simulink library "FPGA_Open_Speech_Tools"  (R2020b)
settings: Solver=VariableStepAuto  StartTime=0.0  StopTime=10.0  RelTol=1e-3
undefined symbols (not defined in the file or in its folder): a, b, c, tableInit
libraries: hdlsllib x159, simulink x26, $bdroot x3
(part 1 of 4)
settings Model: Creator=E. Bailey Galacci  LastModifiedBy=conno
settings SFSimCC: CustomCodeUndefinedFunction=UseInterfaceOnly

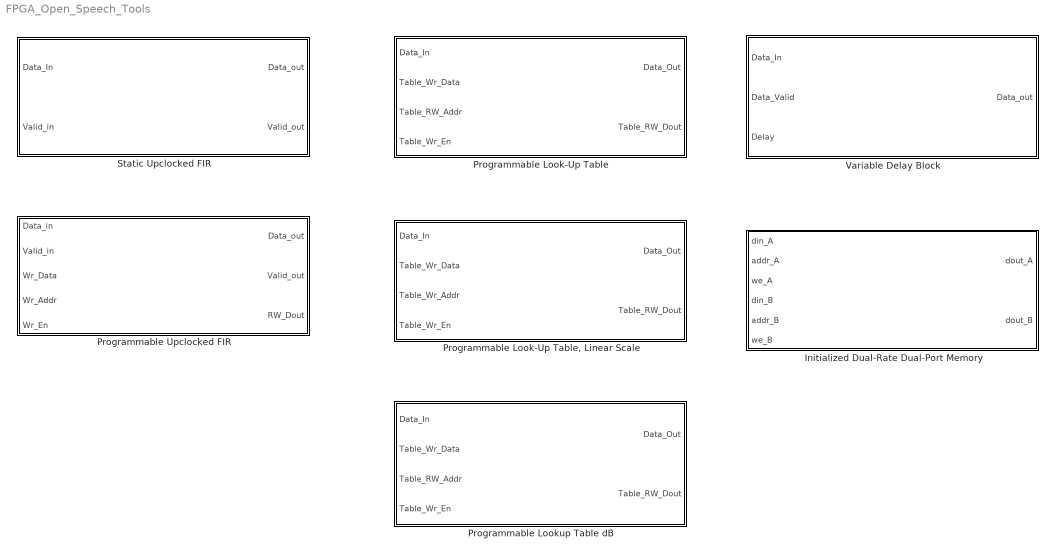
== system FPGA_Open_Speech_Tools ==
  Initialized Dual-Rate Dual-Port Memory : Subsystem  mask(Dual-rate dual-port RAM){ram_size=8, Table_Init=tableInit}
      mask prompts: ram_size "Address port width (2 to 29 bits)"; Table_Init "Table Initialized Values (vector)"
      mask help: This block simulates a dual-clock dual-port RAM with two data output ports. The memory is initialized with values from the Table_Init input vector.
      mask init:
      | hdlblkmask_drdpram;
      mask Help: helpview([docroot '/hdlcoder/helptargets.map'],'HDL_dual_rate_dual_port_ram');
      mask Display:
      | disp(sprintf(['Initialized Dual-Rate \n Dual-Port Memory']));
      | port_label('input',1,'din_A');
      | port_label('input',2,'addr_A');
      | port_label('input',3,'we_A');
      | port_label('input',4,'din_B');
      | port_label('input',5,'addr_B');
      | port_label('input',6,'we_B');
      | port_label('output',1,'dout_A');
      | port_label('output',2,'dout_B');
  Programmable Look-Up Table : Subsystem  mask(Programmable Look-Up Table){tableFnParam=xIn.^0.5, SAVE_TABLE=off, maxInput=1, floorParam=2^-15, errorParam=.1, ERR_DIAG=off, PLOT_TABLE=off, nBitsParam=4, mBitsParam=5, IGOTTHIS=off, W_bits=32, F_bits=28, tableInit=0, binaryOffset=0}
      mask prompts: tableFnParam "Table Represented Function"; SAVE_TABLE "Save Table Input/Output set as .mat"; maxInput "Maximum Input Value"; floorParam "Minimum Input Threshold"; errorParam "Maximum Allowed Error (%)"; ERR_DIAG "Show Error Calculation"; PLOT_TABLE "Show Table Init Plot"; nBitsParam "N_bits"; mBitsParam "M_bits"; IGOTTHIS "Manual Bit Definition Override"; W_bits "Word Bits"; F_bits "Fractional Bits"
      mask help:
      | A hardware-oriented implementation of a lookup table.
      | Provides a fairly resource efficient way to avoid hardware-difficult operations, such as logarithms or square roots.
      | Tables can be initialized on system startup and rewritten during runtime using the Table_Wr lines.
      | Min input cannot be 0, because inputs are pseudo-logarithmically spaced.
      |
      | Input and Output set can be saved as "xIn" and "tableInit" within the file "<path name> init.mat". Input values remain constant
      | until the mask parameters are updated. Table Output values can be reprogrammed during runtime using the Wr_Data, Wr_En and RW_Addr lines.
      mask init:
      | %% PLUT INIT SCRIPT
      | %
      | % This script is a copy of code used in the Programmable Look-Up Table's
      | % init script in the DSP_FPGA_Accelerated_Toolbox.
      | 
      | % Copyright 2020 Flat Earth Inc
      | %
      | % THE SOFTWARE IS PROVIDED "AS IS", WITHOUT WARRANTY OF ANY KIND, EXPRESS OR IMPLIED,
      | % INCLUDING BUT NOT LIMITED TO THE WARRANTIES OF MERCHANTABILITY, FITNESS FOR A PARTICULAR
      | % PURPOSE AND NONINFRINGEMENT. IN NO EVENT SHALL THE AUTHORS OR COPYRIGHT HOLDERS BE LIABLE
      | % FOR ANY CLAIM, DAMAGES OR OTHER LIABILITY, WHETHER IN AN ACTION OF CONTRACT, TORT OR OTHERWISE,
      | % ARISING FROM, OUT OF OR IN CONNECTION WITH THE SOFTWARE OR THE USE OR OTHER DEALINGS IN THE SOFTWARE.
      | %
      | % E. Bailey Galacci
      | % Flat Earth Inc
      | % 985 Technology Blvd
      | % Bozeman, MT 59718
      | % support@flatearthinc.com
      | 
      | % things to display: table size, input bounds, function, accuracy
      | % things to figure out: M_bits, N_bits, Min_val, X_in table, Y_out table,
      | % max_error, ram_size, table_size 
      | 
      | binaryOffset = ceil(log2(maxInput)); % used for binary tricks, as well as identifying input range
      | if(IGOTTHIS)
      |     N_bits = nBitsParam;
      |     M_bits = mBitsParam;
      | else
      |     N_bits = ceil(log2(binaryOffset-log2(floorParam)+1));
      |     % M_bits needs to be defined later, as it must be just enough to meet
      |     % accuracy standards defined by user, with linear interpolation
      |     M_bits = 1; %this will be updated later as needed
      | end
      | 
      | repeatFlag = true;
      | while(repeatFlag)
      |     % Define a N point log2 spaced range of inputs, from 2^(d-(2^N_bits -1)) to almost 2^(d+1), 
      |     % this effectively covers the user defined input range, down to a floor
      |     % value.
      |     xIn = zeros(1, 2^(M_bits+N_bits));
      |     addr = 1;
      |     for NShifts = 2^N_bits-1:-1:0
      |         for M = 0:2^M_bits - 1
      |             xIn(addr) = 2^(binaryOffset-NShifts) + M*2^(binaryOffset-NShifts-M_bits);
      |             addr = addr+1;
      |         end
      |     end
      | 
      |     % use function to define output. note: function must contain input xIn
      |     % within the string to work properly, and the only output of the function
      |     % must be the table values.
      |     tableInit = eval(tableFnParam);
      | 
      |     RAM_SIZE = N_bits+M_bits;
      |     maxVal = 2^binaryOffset+ (2^M_bits -1)*2^(binaryOffset-M_bits);
      |     minVal = 2^(binaryOffset-(2^N_bits-1));
      |     %set_param(gcb,'MaskDisplay',"disp(sprintf('Programmable Look-up Table\nMemory Used = %d samples and coeffs\nClock Rate Needed = %d Hz', FIR_Uprate*2, Max_Rate)); port_label('input',1,'data'); port_label('input',2,'valid'); port_label('input',3,'Wr_Data'); port_label('input',4,'Wr_Addr'); port_label('input',5,'Wr_En'); port_label('output',1,'data'); port_label('output',2,'valid'); port_label('output',3,'RW_Dout');")
      | 
      |     %%%%%%%%%% check and identify error %%%%%%%%%%%
      |     % Define a set of test cases for the lookup table with log spaced points
      |     xTest = logspace(log10(minVal), log10(maxVal), 2^(RAM_SIZE+2));
      |     xTemp = xIn;
      |     xIn = xTest;
      |     % identify the values of the function at xTest
      |     yTest = eval(tableFnParam);
      | 
      |     % move lookup table input values back to xIn
      |     xIn = xTemp;
      | 
      |     % Find lookup addresses for each point in xTest
      |     % Effectively assumes the highest input value, then decreases address until test input is greater than associated table input at that address
      |     addrTest = zeros(1,length(xTest));
      |     for it = 1:length(xTest)
      |         addrTest(it) = 2^RAM_SIZE;
      |         while(xTest(it) < xIn(addrTest(it)) && addrTest(it) ~= 1)   % find the address associated with an input value closest to and below xTest
      |             addrTest(it) = addrTest(it) - 1;
      |         end
      |         if(addrTest(it)==0)
      |             addrTest(it) = 1;
      |         end
      |     end
      | 
      |     % Check for any possible out of bounds errors (handled similarly in hardware)
      |     addrTest(addrTest == 2^RAM_SIZE) = 2^RAM_SIZE -1;
      | 
      |     % Get values for linear interpolation of xIn
      |     xLow  = xIn(addrTest);
      |     xHigh = xIn(addrTest+1);
      | 
      |     % apply point-slope formula to preform linear interpolation for the table readout
      |     yLow  = tableInit(addrTest);
      |     yHigh = tableInit(addrTest+1);
      |     slope  = (yHigh-yLow) ./ (xHigh - xLow);
      |     yInter = slope.*(xTest-xLow)+yLow;
      |     
      |     % percent error: obt-exp / exp
      |     %errorFloor = (yTest-yLow)./yTest;  % w/out linear interpolation
      |     errorInter = (yTest-yInter)./yTest; % w/ linear interpolation
      |     maxErr = max(abs(errorInter));
      |     %check while loop condition
      |     if(IGOTTHIS) 
      |         repeatFlag = false;
      |     else
      |         if(100*maxErr <= abs(errorParam))
      |             repeatFlag = false;
      |         else
      | %             if(ERR_DIAG)
      | %                 f = msgbox(sprintf('Err = %.2d, M_bits = %d', 100*maxErr, M_bits),'Configuring PLUT','replace');
      | %             end
      |             
      |             % make table larger to increase accuracy. M_bits can increase
      |             % by more than 1 to save loops if error is far outside bounds
      |             if(100*maxErr > 8*errorParam)
      |                 M_bits = M_bits+3;
      |             elseif(100*maxErr > 4*errorParam)
      |                 M_bits = M_bits+2;
      |             else
      |                 M_bits = M_bits+1;
      |             end
      |         end
      |     end
      | end%end while loop
      | % prinout graph of table values and error test
      | if(ERR_DIAG)
      |     figure(1); 
      |     f = msgbox(sprintf('%s\nErr = %.2d %%, Ram Size = %d bits  (2 by %d by %d)\n Address Width: %d, N_bits: %d, M_bits: %d', gcb, 100*maxErr, 2*2^RAM_SIZE*W_bits, 2^RAM_SIZE, W_bits, RAM_SIZE, N_bits, M_bits), sprintf('PLUT INIT: %s', gcb),'replace');
      |     subplot(2,1,1); semilogx(xTest,yInter, xTest,yTest,xIn,tableInit,'k*'); title('Output Values over Input Range'); xlabel('Inputs'); ylabel('Outputs'); legend('Interpolated Results','Ideal','Table Points');
      |     subplot(2,1,2); semilogx(xTest,100*errorInter); title('Error of Output over Input Range'); xlabel('Inputs'); ylabel('Percent Error');
      | end
      | 
      | % Some testing variables. Uncomment if desired.
      | %maxFloorErrTot = max(maxFloorErr);
      | %maxInterErrTot = max(maxInterErr);
      | 
      | % Plot the LUT's inital table set
      | if(PLOT_TABLE)
      |     % Handle String errors? 
      |     figure(2); semilogx(xIn,tableInit, 'k*'); title(sprintf('Table Initialized Function: %s', tableFnParam),'Interpreter','none');
      | end 
      | % Save Input and Output set to a .mat file
      | if(SAVE_TABLE)
      |     fileName = [gcb '_init'];
      |     fileName(fileName == '/') = '_'; % Replace slashes with underscores
      |     address = 0:(2^RAM_SIZE)-1;
      |     save(fileName, 'xIn', 'address', 'tableInit');
      | end
      | set_param(gcb,'MaskDisplay',"disp(sprintf(['Programmable Look-Up Table\nMemory Used: %d bits, Address Width: %d\n' tableFnParam ': %.2d <= x <= %.2d\n Maximum Error: %.2d %%'], 2*2^RAM_SIZE*W_bits, RAM_SIZE, minVal, maxVal, 100*maxErr)); port_label('input',1,'Data_In'); port_label('input',2,'Table_Wr_Data'); port_label('input',3,'Table_RW_Addr'); port_label('input',4,'Table_Wr_En'); port_label('output',1,'Data_Out'); port_label('output',2,'Table_RW_Dout');")
      mask Help:
      | A hardware-oriented implementation of a lookup table.
      | Provides a fairly resource efficient way to avoid hardware-difficult operations, such as logarithms or square roots.
      | Tables can be initialized on system startup and rewritten during runtime using the Table_Wr lines.
      | Min input cannot be 0, because inputs are pseudo-logarithmically spaced.
      | 
      | Input and Output set can be saved as "xIn" and "tableInit" within the file "<path name> init.mat". Input values remain constant
      | until the mask parameters are updated. Table Output values can be reprogrammed during runtime using the Wr_Data, Wr_En and RW_Addr lines.
      | 
      | Uses pseudo-logarithmic spacing of inputs for maximum accuracy in non-linear functions, as well as linear interpolation between points to further increase accuracy. Because of this, it is assumed that function input is unsigned. If this is undesired, a second table would need to be implemented to cover negative values, or some other solution outside the block.
      | 
      | Capable of automatically determining required table size to meet a given accuracy requirement within the entire data range, or can be manually set to a specific size with M_bits and N_bits. N_bits determines the data range as a power of 1/2 of the maximum input. M_bits determines the number of bits in the address used to increase function precision, by increasing the number of points stored between each log2 spaced input point.
      | 
      | 
      | 
      | ------------------
      | Mask Parameters
      | ------------------
      | 
      | Table Represented Function:
      |   Function to estimate using the lookup table. Must contain the variable "X_in" as an input to a function, or as a variable within the executable code string, as this is used in the Initialization code to evaluate the function. If a function, that function must also have a single output which will define the values to fill the table with given input value X_in.
      | 
      | Save Table Input/Output set as .mat
      |   If asserted, the table's inputs and outputs will be saved in a .mat file named "<path name>_init.mat". By loading this, it is possible to see all precalculated points of the look-up table. This is especially useful when trying to reprogram the table, as all input points are shown along with their associated addresses.
      | 
      | --Table Parameters--
      |   Maximum Input Value:
      |     The maximum input value the table should be expected to represent. If the input value is greater than this parameter's nearest higher power of 2, the table will output the value for the highest input.
      | 
      | --Define Input Threshold and Accuracy Tab--
      |   Minimum Input Threshold:
      |     The minimum input to recognize by the table. If the input value is less than this parameter's the nearest lower power of 2, the table will output the value for the lowest input.
      | 
      |   Maximum Allowed Error (%):
      |     The amount of percent error allowed by the table. Used by the init script to identify the size of the table required to meet this parameter. This is found by testing a set of examples 4 times larger than the table set, therefore it is possible on rare occasion for some points to exceed this error. Decreasing this will increase the memory required for the table, but increase precision.
      | 
      |   Show Error Calculation:
      |     When asserted, the block will show a figure of the error calculation and a pop-up detailing the amount of memory used, size of the RAM allocated, and maximum error.
      | 
      |   Show Table Init Plot:
      |     When asserted, the block will show a figure of the table's initialized values.
      | 
      | --Define Address Space Manually Tab--
      |   N_bits:
      |     Only used when Manual Bit Definition Override is asserted.
      |     The width of the address dedicated to breadth of valid data. Increasing this will cause the table to recognize smaller numbers (by increasing the size of the Leading Zero Counter's output)  at the cost of memory used, and more logic required in the LZC.
      |   M_bits:
      |     Only used when Manual Bit Definition Override is asserted.
      |     The width of the address dedicated to depth of valid data. Increasing this will cause more bits of the input to be considered as part of the address after the Leading Zero Counter, increasing precision at the cost of memory.
      | 
      |   Manual Bit Definition Override:
      |     Checking this box will skip automatic size definition of Leading Zero Counter and precision bit size. Use with caution, as percent error will not be guaranteed with this setting on. Read the formal documentation for more details, kept within the file structure this library is stored in.
      | 
      | 
      | --Data Parameters dropdown--
      | Word Bits:
      |   Size of fixed point word of both the input signal and table memory.
      | 
      | Fractional Bits:
      |   Number of fractional bits in the fixed point word of both the input signal and table memory.
      | 
      | ----------
      | Block I/O
      | ----------
      | INPUTS:
      | 
      | --Data_In--
      |   Input signal to be looked-up. Expected size fixdt(0,Word Bits, Fractional Bits).
      | 
      | --Table_Wr_Data-- % Table Write Data
      |   Data to write to the table, in location Table_RW_Addr, when Table_Wr_En is asserted. Expected size fixdt(0,Word Bits, Fractional Bits).
      | 
      | --Table_RW_Addr-- % Table Read/Write Address
      |   The location within the table to read or overwrite. Expected size changes based on the function and allowed error as initialized, and is shown on the Mask Label as RAM Width, or by checking the "Show Error Calculation" button as RAM Width.
      |   There is an internal check that will correct a signal of the wrong size to the correct address size, but it may be useful to know the X values associated with table output at any given address. Using the "Save Table Input/Output as .mat" option will save the entire set of initialized inputs and outputs along with their associated addresses.
      |   For a full explanation on how xIn is derived, see the formal documentation contained within the file structure this library is stored in.
      | 
      | --Table_Wr_En-- % Table Write Enable
      |   Boolean. If this line is asserted, address Table_RW_Addr will be overwritten with data Table_Wr_Data.
      | 
      | 
      | OUTPUTS:
      | --Data_Out--
      |   Output data of the table. Size fixdt(1,Word Bits, Fractional Bits).
      | 
      | --Table_RW_Dout-- % Table Read/Write Data Out
      |   Outputs the data currently within address Table_RW_Addr (after writing if Table_Wr_En is asserted). Size fixdt(1, Word Bits, Fractional Bits).
      mask DialogControl Control2_copy Prompt: Must be a function of "xIn" to get table values
      mask DialogControl Container3 Prompt: Table Parameters
      mask DialogControl Container5 Prompt: Define Input Threshold and Accuracy
      mask DialogControl Container7 Prompt: Define Address Space Manually
      mask DialogControl Control2 Prompt: See Documentation for details
      mask DialogControl Container9 Prompt: Data Parameters
      mask Display: disp(sprintf(['Programmable Look-Up Table\nMemory Used: %d bits, Address Width: %d\n' tableFnParam ': %.2d <= x <= %.2d\n Maximum Error: %.2d %%'], 2*2^RAM_SIZE*W_bits, RAM_SIZE, minVal, maxVal, 100*maxErr)); port_label('input',1,'Data_In'); port_label('input',2,'Table_Wr_Data'); port_label('input',3,'Table_RW_Addr'); port_label('input',4,'Table_Wr_En'); port_label('output',1,'Data_Out'); port_label('output',2,'Table_RW_Dout');
  "Programmable Look-Up Table, Linear Scale" : Subsystem  mask(Programmable Look-Up Table){tableFnParam=sin(xIn), SAVE_TABLE=off, errorParam=.1, ERR_DIAG=off, PLOT_TABLE=off, ADDR_W_MANUAL=4, IGOTTHIS=off, W_bits=32, F_bits=28, isSigned=on, tableInit=0}
      mask prompts: tableFnParam "Table Represented Function"; SAVE_TABLE "Save Table Input/Output set as .mat"; errorParam "Maximum Allowed Error (+/-)"; ERR_DIAG "Show Error Calculation"; PLOT_TABLE "Show Table Init Plot"; ADDR_W_MANUAL "Address Width"; IGOTTHIS "Manual Bit Definition Override"; W_bits "Word Bits"; F_bits "Fractional Bits"; isSigned "Data Signed?"
      mask help:
      | A hardware-oriented implementation of a lookup table.
      | Provides a fairly resource efficient way to avoid hardware-difficult operations, such as logarithms or square roots.
      | Tables can be initialized on system startup and rewritten during runtime using the Table_Wr lines.
      mask init:
      | %% LINEAR PLUT INIT SCRIPT
      | 
      | % Copyright 2020 Flat Earth Inc
      | %
      | % THE SOFTWARE IS PROVIDED "AS IS", WITHOUT WARRANTY OF ANY KIND, EXPRESS OR IMPLIED,
      | % INCLUDING BUT NOT LIMITED TO THE WARRANTIES OF MERCHANTABILITY, FITNESS FOR A PARTICULAR
      | % PURPOSE AND NONINFRINGEMENT. IN NO EVENT SHALL THE AUTHORS OR COPYRIGHT HOLDERS BE LIABLE
      | % FOR ANY CLAIM, DAMAGES OR OTHER LIABILITY, WHETHER IN AN ACTION OF CONTRACT, TORT OR OTHERWISE,
      | % ARISING FROM, OUT OF OR IN CONNECTION WITH THE SOFTWARE OR THE USE OR OTHER DEALINGS IN THE SOFTWARE.
      | %
      | % E. Bailey Galacci
      | % Flat Earth Inc
      | % 985 Technology Blvd
      | % Bozeman, MT 59718
      | % support@flatearthinc.com
      | 
      | % things to display: table size, floor input?, max input, accuracy
      | % things to figure out: M_bits, N_bits, Min_val, X_in table, Y_out table,
      | % maxError, RAM_SIZE, table size 
      | 
      | if(IGOTTHIS)
      |     N_bits = ADDR_W_MANUAL;
      | else
      |     N_bits = 4;
      |     % N_bits will likely need to be updated later, until table is large enough to meet
      |     % accuracy standards defined by user
      | end;
      | 
      | repeatFlag = true;
      | while(repeatFlag)
      |     % Define a 2^N point log2 spaced range of inputs, from 2^(d-(2^N_bits -1)) to almost 2^(d+1), 
      |     % this effectively covers the user defined input range, down to a floor
      |     % value.
      |     % Signed vs Unsigned: If signed, treat word size as 1 smaller for max and
      |     % min inputs
      |     % Signed: 
      |     % smallest table input: -2^(W-1-F), 2's compliment, "[1, zeros(1,N-1)]"
      |     % step size: 2^(W-F-N)
      |     % largest table input: 2^(W-1-F) - 2^(W-F-N), smallest number but positive
      |     % and minus 1 step size, "[0, ones(1,N-1)]"
      |     % Unsigned: 
      |     % smallest table input: 0
      |     % step size: 2^(W-F-N)
      |     % largest table input: 2^(W-1-F) - 2^(W-F-N), smallest number but positive
      |     % and minus 1 step size, "[ones(1,N)]"
      |     if(isSigned)
      |         xIn = -2^(W_bits-1-F_bits) : 2^(W_bits-F_bits-N_bits) : 2^(W_bits-1-F_bits) - 2^(W_bits-F_bits-N_bits);
      |     else
      |         xIn = 0 : 2^(W_bits-F_bits-N_bits) : 2^(W_bits-F_bits) - 2^(W_bits-F_bits-N_bits);
      |     end
      | 
      |     % use function to define output. note: function must contain input xIn
      |     % within the string to work properly, and the only output of the function
      |     % must be Y_out.
      |     tableInit = eval(tableFnParam);
      | 
      |     RAM_SIZE = N_bits;
      |     maxVal = xIn(end);
      |     minVal = xIn(1);
      |     %set_param(gcb,'MaskDisplay',"disp(sprintf('Programmable Look-up Table\nMemory Used = %d samples and coeffs\nClock Rate Needed = %d Hz', FIR_Uprate*2, Max_Rate)); port_label('input',1,'data'); port_label('input',2,'valid'); port_label('input',3,'Wr_Data'); port_label('input',4,'Wr_Addr'); port_label('input',5,'Wr_En'); port_label('output',1,'data'); port_label('output',2,'valid'); port_label('output',3,'RW_Dout');")
      | 
      |     %%%%%%%%%% check and identify error %%%%%%%%%%%
      |     % Make some values for an "ideal" lookup table with lin spaced points
      |     if(isSigned)
      |         xTest = -2^(W_bits-1-F_bits) : 2^(W_bits-F_bits-N_bits-2) : 2^(W_bits-1-F_bits) - 2^(W_bits-F_bits-N_bits);
      |     else
      |         xTest = 0 : 2^(W_bits-F_bits-N_bits-2) : 2^(W_bits-F_bits) - 2^(W_bits-F_bits-N_bits);
      |     end
      |     xTemp = xIn;
      |     xIn = xTest;
      |     % identify the values of the function at xTest
      |     yTest = eval(tableFnParam);
      | 
      |     % Return table input set to xIn (already have xTemp)
      |     xIn = xTemp;
      | 
      |     % Find lookup addresses for each point in xTest
      |     addrTest = zeros(1,length(xTest));
      |     for it = 1:length(xTest)
      |         addrTest(it) = 2^RAM_SIZE;
      |         while(xTest(it) < xIn(addrTest(it)) && addrTest(it) ~= 1)
      |             addrTest(it) = addrTest(it) - 1;
      |         end
      |         if(addrTest(it)==0) %% sanity check for out of bounds results
      |             addrTest(it) = 1;
      |         end
      |     end
      |     
      |     yLow = tableInit(addrTest);
      | 
      |     % Check for any possible out of bounds errors (handled similarly in
      |     % hardware)
      |     addrTest(addrTest == 2^RAM_SIZE) = 2^RAM_SIZE -1;
      | 
      |     
      |     % absolute error: abs(obt-exp)
      |     errorFloor = abs(yTest-yLow);
      |     NAN_CLEANUP = isnan(errorFloor);
      |     errorFloor(NAN_CLEANUP) = 0;
      |     %errorInter = (Y_out_Ideal-y_inter)./Y_out_Ideal;
      |     %maxFloorErr(ix) = 100*max(abs(errorFloor(ix, 2870:9839)));
      |     %maxInterErr(ix) = 100*max(abs(errorInter(ix, 2870:9839)));
      |     maxErr = max(abs(errorFloor));
      |     
      |     %check while loop condition
      |     if(IGOTTHIS) 
      |         repeatFlag = false;
      |     end
      |     
      |     if(maxErr <= abs(errorParam) || N_bits > W_bits)
      |         repeatFlag = false;
      |     else
      | %        if(ERR_DIAG)
      | %            f = msgbox(sprintf('Err = %.2d, N_bits = %d', maxErr, N_bits),'Configuring PLUT','replace');
      | %        end
      |         
      |         % make table larger to increase accuracy
      |         if(maxErr > abs(errorParam))
      |             N_bits = N_bits+1;
      |         end
      |     end
      | end%end while loop
      | 
      | % Plot the LUT's inital table set
      | if(PLOT_TABLE)
      |     % Handle String errors? 
      |     figure(2); semilogx(xIn,tableInit, 'k*'); title(sprintf('Table Initialized Function: %s', tableFnParam),'Interpreter','none');
      | end 
      | 
      | % printout graph of table values and error test
      | if(ERR_DIAG)
      |     figure(1); 
      |     f = msgbox(sprintf('Err = +/- %.2d, Ram Size = %d bits  (%d by %d)', maxErr, 2^RAM_SIZE*W_bits, 2^RAM_SIZE, W_bits),gcb,'replace');
      |     subplot(2,1,1); plot(xTest,yLow, xTest,yTest,xIn,tableInit,'k*'); title('Output Values over Input Range'); xlabel('Inputs'); ylabel('Outputs'); legend('Table Results','Ideal','Table Points');
      |     subplot(2,1,2); plot(xTest, errorFloor); title('Error of Output over Input Range'); xlabel('Inputs'); ylabel('Absolute Error');
      | end
      | 
      | if(isSigned) % setup for 2's compliment
      |     tableInit = [tableInit(2^(N_bits-1)+1:end) , tableInit(1:2^(N_bits-1))];
      |     xInInit = [xIn(2^(N_bits-1)+1:end), xIn(1:2^(N_bits-1))];
      | else
      |     tableInit = tableInit;
      |     xInInit = xIn;
      | end
      | 
      | % Save Input and Output set to a .mat file
      | if(SAVE_TABLE)
      |     fileName = [gcb '_init'];
      |     fileName(fileName == '/') = '_'; % Replace slashes with underscores
      |     address = 0:(2^RAM_SIZE)-1;
      |     save(fileName, 'xInInit', 'address', 'tableInit');
      | end
      | 
      | set_param(gcb,'MaskDisplay',"disp(sprintf(['Programmable Look-Up Table\nMemory Used = %d bits, Address Width: %d\n' tableFnParam ': %d <= x <= %d \n Maximum Error: +/-%.2d'], 2^RAM_SIZE*W_bits, RAM_SIZE, minVal, maxVal, maxErr)); port_label('input',1,'Data_In'); port_label('input',2,'Table_Wr_Data'); port_label('input',3,'Table_RW_Addr'); port_label('input',4,'Table_Wr_En'); port_label('output',1,'Data_Out'); port_label('output',2,'Table_RW_Dout');")
      mask Help:
      | A hardware-oriented implementation of a lookup table.
      | Provides a fairly resource efficient way to avoid hardware-difficult operations, such as logarithms or square roots.
      | Tables can be initialized on system startup and rewritten during runtime using the Table_Wr lines.
      | 
      | 
      | Capable of automatically determining required table size to meet a given accuracy requirement within the entire data range, or can be manually set to a specific size with N_bits. Data Range is determined by the word size and fractional bit size of data entering the PLUT.
      | 
      | 
      | 
      | ------------------
      | Mask Parameters
      | ------------------
      | 
      | Table Represented Function:
      |   Function to estimate using the lookup table. Must contain the variable "X_in" as an input to a function, or as a variable within the executable code string, as this is used in the Initialization code to evaluate the function. If a function, that function must also have a single output which will define the values to fill the table with given input value X_in.
      | 
      | Save Table Input/Output set as .mat
      |   If asserted, the table's inputs and outputs will be saved in a .mat file named "<path name>_init.mat". By loading this, it is possible to see all precalculated points of the look-up table. This is especially useful when trying to reprogram the table, as all input points are shown along with their associated addresses.
      | 
      | --Table Parameters--
      |   Maximum Input Value:
      |     The maximum input value the table should be expected to represent. This is based on the data range of the fixed point word size and fractional size, and adjusted if the data is signed.
      | 
      | --Define Input Range and Accuracy Tab--
      |   Maximum Allowed Error (+/-):
      |     The amount of absolute error allowed by the table. Used by the init script to identify the size of the table required to meet this parameter. This is found by testing a set of examples 4 times larger than the table set, therefore it is possible on rare occasion for some points to exceed this error. Decreasing this will increase the memory required for the table, but increase precision.
      | 
      |   Show Error Calculation:
      |     When asserted, the block will show a figure of the error calculation and a pop-up detailing the amount of memory used, size of the RAM allocated, and maximum error.
      | 
      |   Show Table Init Plot:
      |     When asserted, the block will show a figure of the table's initialized values.
      | 
      | --Define Address Space Manually Tab--
      |   Address Width:
      |     Only used when Manual Bit Definition Override is asserted.
      |     The width of the address dedicated to depth of valid data.  Increasing this will cause more bits of the input to be considered as part of the address, increasing precision at the cost of memory.
      | 
      |   Manual Bit Definition Override:
      |     Checking this box will skip automatic size definition of precision bit size. Use with caution, as absolute error will not be guaranteed with this setting on. Read the formal documentation for more details, kept within the file structure this library is stored in.
      | 
      | 
      | --Data Parameters dropdown--
      | Word Bits:
      |   Size of fixed point word of both the input signal and table memory.
      | 
      | Fractional Bits:
      |   Number of fractional bits in the fixed point word of both the input signal and table memory.
      | 
      | Data Signed?
      |   Check if data is signed. Adjusts table's values and readout if data is signed.
      | 
      | ----------
      | Block I/O
      | ----------
      | INPUTS:
      | 
      | --Data_In--
      |   Input signal to be looked-up. Expected size fixdt(isSigned,Word Bits, Fractional Bits).
      | 
      | --Table_Wr_Data-- % Table Write Data
      |   Data to write to the table, in location Table_RW_Addr, when Table_Wr_En is asserted. Expected size fixdt(isSigned,Word Bits, Fractional Bits).
      | 
      | --Table_RW_Addr-- % Table Read/Write Address
      |   The location within the table to read or overwrite. Expected size changes based on the function and allowed error as initialized, and is shown on the Mask Label as RAM Width, or by checking the "Show Error Calculation" button as RAM Width.
      |   There is an internal check that will correct a signal of the wrong size to the correct address size, but it may be useful to know the X values associated with table output at any given address. Using the "Save Table Input/Output as .mat" option will save the entire set of initialized inputs and outputs along with their associated addresses.
      |   For a full explanation on how xIn is derived, see the formal documentation contained within the file structure this library is stored in.
      | 
      | --Table_Wr_En-- % Table Write Enable
      |   Boolean. If this line is asserted, address Table_RW_Addr will be overwritten with data Table_Wr_Data.
      | 
      | 
      | OUTPUTS:
      | --Data_Out--
      |   Output data of the table. Size fixdt(isSigned,Word Bits, Fractional Bits).
      | 
      | --Table_RW_Dout-- % Table Read/Write Data Out
      |   Outputs the data currently within address Table_RW_Addr (after writing if Table_Wr_En is asserted). Size fixdt(isSigned, Word Bits, Fractional Bits).
      mask DialogControl Control2_copy Prompt: Must be a function of xIn to get yOut
      mask DialogControl Container3 Prompt: Table Parameters
      mask DialogControl Container5 Prompt: Define Input Range and Accuracy
      mask DialogControl Container7 Prompt: Define Address Space Manually
      mask DialogControl Control2 Prompt: See Documentation for details
      mask DialogControl Container9 Prompt: Data Parameters
      mask Display: disp(sprintf(['Programmable Look-Up Table\nMemory Used = %d bits, Address Width: %d\n' tableFnParam ': %d <= x <= %d \n Maximum Error: +/-%.2d'], 2^RAM_SIZE*W_bits, RAM_SIZE, minVal, maxVal, maxErr)); port_label('input',1,'Data_In'); port_label('input',2,'Table_Wr_Data'); port_label('input',3,'Table_RW_Addr'); port_label('input',4,'Table_Wr_En'); port_label('output',1,'Data_Out'); port_label('output',2,'Table_RW_Dout');
  Programmable Lookup Table dB : Subsystem  mask(Programmable Look-Up Table){tableFnParam=10.*log10(2500000000.*xIn), SAVE_TABLE=off, maxInput=1, floorParam=2^-31, errorParam=1, ERR_DIAG=off, PLOT_TABLE=off, nBitsParam=5, mBitsParam=4, IGOTTHIS=off, W_bits=40, F_bits=32, tableInit=0, binaryOffset=0}
      mask prompts: tableFnParam "Table Represented Function"; SAVE_TABLE "Save Table Input/Output set as .mat"; maxInput "Maximum Input Value"; floorParam "Minimum Input Threshold"; errorParam "Maximum Allowed Error (%)"; ERR_DIAG "Show Error Calculation"; PLOT_TABLE "Show Table Init Plot"; nBitsParam "N_bits"; mBitsParam "M_bits"; IGOTTHIS "Manual Bit Definition Override"; W_bits "Word Bits"; F_bits "Fractional Bits"
      mask help:
      | A hardware-oriented implementation of a lookup table.
      | Provides a fairly resource efficient way to avoid hardware-difficult operations, such as logarithms or square roots.
      | Tables can be initialized on system startup and rewritten during runtime using the Table_Wr lines.
      | Min input cannot be 0, because inputs are pseudo-logarithmically spaced.
      |
      | Input and Output set can be saved as "xIn" and "tableInit" within the file "<path name> init.mat". Input values remain constant
      | until the mask parameters are updated. Table Output values can be reprogrammed during runtime using the Wr_Data, Wr_En and RW_Addr lines.
      mask init: same as FPGA_Open_Speech_Tools/Programmable Look-Up Table
      mask Help:
      | A hardware-oriented implementation of a lookup table.
      | Provides a fairly resource efficient way to avoid hardware-difficult operations, such as logarithms or square roots.
      | Tables can be initialized on system startup and rewritten during runtime using the Table_Wr lines.
      | Min input cannot be 0, because inputs are pseudo-logarithmically spaced.
      | 
      | Input and Output set can be saved as "xIn" and "tableInit" within the file "<path name> init.mat". Input values remain constant
      | until the mask parameters are updated. Table Output values can be reprogrammed during runtime using the Wr_Data, Wr_En and RW_Addr lines.
      | 
      | Uses pseudo-logarithmic spacing of inputs for maximum accuracy in non-linear functions, as well as linear interpolation between points to further increase accuracy. Because of this, it is assumed that function input is unsigned. If this is undesired, a second table would need to be implemented to cover negative values, or some other solution outside the block.
      | 
      | Capable of automatically determining required table size to meet a given accuracy requirement within the entire data range, or can be manually set to a specific size with M_bits and N_bits. N_bits determines the data range as a power of 1/2 of the maximum input. M_bits determines the number of bits in the address used to increase function precision, by increasing the number of points stored between each log2 spaced input point.
      | 
      | 
      | 
      | ------------------
      | Mask Parameters
      | ------------------
      | 
      | Table Represented Function:
      |   Function to estimate using the lookup table. Must contain the variable "X_in" as an input to a function, or as a variable within the executable code string, as this is used in the Initialization code to evaluate the function. If a function, that function must also have a single output which will define the values to fill the table with given input value X_in.
      | 
      | Save Table Input/Output set as .mat
      |   If asserted, the table's inputs and outputs will be saved in a .mat file named "<path name>_init.mat". By loading this, it is possible to see all precalculated points of the look-up table. This is especially useful when trying to reprogram the table, as all input points are shown along with their associated addresses.
      | 
      | --Table Parameters--
      |   Maximum Input Value:
      |     The maximum input value the table should be expected to represent. If the input value is greater than this parameter's nearest higher power of 2, the table will output the value for the highest input.
      | 
      | --Define Input Threshold and Accuracy Tab--
      |   Minimum Input Threshold:
      |     The minimum input to recognize by the table. If the input value is less than this parameter's the nearest lower power of 2, the table will output the value for the lowest input.
      | 
      |   Maximum Allowed Error (%):
      |     The amount of percent error allowed by the table. Used by the init script to identify the size of the table required to meet this parameter. This is found by testing a set of examples 4 times larger than the table set, therefore it is possible on rare occasion for some points to exceed this error. Decreasing this will increase the memory required for the table, but increase precision.
      | 
      |   Show Error Calculation:
      |     When asserted, the block will show a figure of the error calculation and a pop-up detailing the amount of memory used, size of the RAM allocated, and maximum error.
      | 
      |   Show Table Init Plot:
      |     When asserted, the block will show a figure of the table's initialized values.
      | 
      | --Define Address Space Manually Tab--
      |   N_bits:
      |     Only used when Manual Bit Definition Override is asserted.
      |     The width of the address dedicated to breadth of valid data. Increasing this will cause the table to recognize smaller numbers (by increasing the size of the Leading Zero Counter's output)  at the cost of memory used, and more logic required in the LZC.
      |   M_bits:
      |     Only used when Manual Bit Definition Override is asserted.
      |     The width of the address dedicated to depth of valid data. Increasing this will cause more bits of the input to be considered as part of the address after the Leading Zero Counter, increasing precision at the cost of memory.
      | 
      |   Manual Bit Definition Override:
      |     Checking this box will skip automatic size definition of Leading Zero Counter and precision bit size. Use with caution, as percent error will not be guaranteed with this setting on. Read the formal documentation for more details, kept within the file structure this library is stored in.
      | 
      | 
      | --Data Parameters dropdown--
      | Word Bits:
      |   Size of fixed point word of both the input signal and table memory.
      | 
      | Fractional Bits:
      |   Number of fractional bits in the fixed point word of both the input signal and table memory.
      | 
      | ----------
      | Block I/O
      | ----------
      | INPUTS:
      | 
      | --Data_In--
      |   Input signal to be looked-up. Expected size fixdt(0,Word Bits, Fractional Bits).
      | 
      | --Table_Wr_Data-- % Table Write Data
      |   Data to write to the table, in location Table_RW_Addr, when Table_Wr_En is asserted. Expected size fixdt(0,Word Bits, Fractional Bits).
      | 
      | --Table_RW_Addr-- % Table Read/Write Address
      |   The location within the table to read or overwrite. Expected size changes based on the function and allowed error as initialized, and is shown on the Mask Label as RAM Width, or by checking the "Show Error Calculation" button as RAM Width.
      |   There is an internal check that will correct a signal of the wrong size to the correct address size, but it may be useful to know the X values associated with table output at any given address. Using the "Save Table Input/Output as .mat" option will save the entire set of initialized inputs and outputs along with their associated addresses.
      |   For a full explanation on how xIn is derived, see the formal documentation contained within the file structure this library is stored in.
      | 
      | --Table_Wr_En-- % Table Write Enable
      |   Boolean. If this line is asserted, address Table_RW_Addr will be overwritten with data Table_Wr_Data.
      | 
      | 
      | OUTPUTS:
      | --Data_Out--
      |   Output data of the table. Size fixdt(1,Word Bits, Fractional Bits).
      | 
      | --Table_RW_Dout-- % Table Read/Write Data Out
      |   Outputs the data currently within address Table_RW_Addr (after writing if Table_Wr_En is asserted). Size fixdt(1, Word Bits, Fractional Bits).
      mask DialogControl Control2_copy Prompt: Must be a function of "xIn" to get table values
      mask DialogControl Container3 Prompt: Table Parameters
      mask DialogControl Container5 Prompt: Define Input Threshold and Accuracy
      mask DialogControl Container7 Prompt: Define Address Space Manually
      mask DialogControl Control2 Prompt: See Documentation for details
      mask DialogControl Container9 Prompt: Data Parameters
      mask Display: disp(sprintf(['Programmable Look-Up Table\nMemory Used: %d bits, Address Width: %d\n' tableFnParam ': %.2d <= x <= %.2d\n Maximum Error: %.2d %%'], 2*2^RAM_SIZE*W_bits, RAM_SIZE, minVal, maxVal, 100*maxErr)); port_label('input',1,'Data_In'); port_label('input',2,'Table_Wr_Data'); port_label('input',3,'Table_RW_Addr'); port_label('input',4,'Table_Wr_En'); port_label('output',1,'Data_Out'); port_label('output',2,'Table_RW_Dout');
  Programmable Upclocked FIR : Subsystem  mask(Programmable Upclocked FIR){b_k=[0.5,0.5], Ts=1/48000, Ts_system=1/96000, rotationDelay=0, W_bits=32, F_bits=28, maxRate=48000}
      mask prompts: b_k "B_k coefficients (vector)"; Ts "Sample Time"; Ts_system "System Time"; rotationDelay "Added Delay"; W_bits "Fixed Point Word Size"; F_bits "Fixed Point Frac Size"
      mask help:
      | This block is designed for a hardware implementation of an FIR filter. The main advantage is resource sharing by using a single multiply/add at an increased clock rate to multiply the b_k coefficients and sum the results.
      | The cost is a slightly increased amount of RAM used and the requirement that the system can run at data_rate*b_k_length, where b_k_length is rounded up to the nearest power of 2. The gains over a traditional FIR are a vastly decreased latency and logic resource usage.
      mask init:
      | FIR_SIZE = ceil(log2(length(b_k)+rotationDelay));
      | FIR_UPRATE = 2^FIR_SIZE;
      | firCoeff = zeros(1,FIR_UPRATE);
      | firCoeff(1:length(b_k)) = b_k;
      | maxRate = 1/(Ts/FIR_UPRATE);
      | 
      | set_param(gcb,'MaskDisplay',"disp(sprintf('Programmable Clock-Accelerated FIR\nMemory Used = %d bits \nFIR Length: %d \nClock Rate Needed = %d Hz', 2*2^FIR_SIZE*W_bits, 2^FIR_SIZE, maxRate)); port_label('input',1,'data'); port_label('input',2,'valid'); port_label('input',3,'Wr_Data'); port_label('input',4, 'RW_Addr'); port_label('input',5,'Wr_En'); port_label('output',1,'data'); port_label('output',2,'valid'); port_label('output',3,'RW_Dout');")
      mask Help:
      | This block is designed for a hardware implementation of an FIR filter. The main advantage is resource sharing by using a single multiply/add at an increased clock rate to multiply the b_k coefficients and sum the results.
      | The cost is a slightly increased amount of RAM used and the requirement that the system can run at data_rate*b_k_length, where b_k_length is rounded up to the nearest power of 2. The gains over a traditional FIR are a vastly decreased latency and logic resource usage.
      | 
      | An "Added Delay" option is included as a way to save resources when delaying the filtered signal. The b_k RAM is padded with 0s to round length up to a power of 2. Therefore, many faster cycles are completely uneccessary. Since many b_k's are 0, they can be rotated to align with inputs starting before the most recent, effectively delaying the output signal with 0 extra resources used. Useful for things like realigning a signal after multi-channel processing, or any other reason to delay the signal. If Added Delay would cause rotation to read from undesired coefficients (not 0), on startup the system will automatically increase the size of the table. This doubles the RAM used, so if using a b_k length at or near a power of 2, or if a very long delay is required, this may not be the most efficient option.
      | 
      | B_k's are defined on system start-up and can be changed during runtime through the Wr_Data, Wr_Addr, and Wr_En signals.
      | B_k's can be ready using the Wr_Addr, Wr_En set to 0, sent out to the RW_Dout line.
      | 
      | ------------------
      | Mask Parameters
      | ------------------
      | 
      | B_k coefficients:
      |   FIR filter coefficients
      | Sample Time:
      |   Amount of time between valid pulses, when the input signal needs to be recognized.
      | System Time:
      |   Amount of time between system clock cycles. Can be the same as Sample Time if Valid_in is always 1.
      | Added Delay:
      |   Adds a N-sample delay to the output. Check Documentation Description for details.
      | Fixed Point Word/Frac Size:
      |   Word and Fractional bit size of input and table data type. Data input and b_k's are assumed to be the same data type.
      | 
      | ----------
      | Block I/O
      | ----------
      | 
      | Data_in:
      |   Input signal to be processed. Can be of any rate a direct multiple of "Sample rate". Signed Fixed Point of size "Fixed Point Word Size".
      | Valid_in:
      |  Trigger to show input signal should be written to signal memory of FIR RAM. Active high. Boolean.
      | Wr_Data:
      |   Data to write to B_k at address Wr_Addr if Wr_En is set to 1. Data type overwritten to match input signal type.
      | Wr_Addr:
      |   Location in table to write or read B_k table. Starts at 0 and ends at 2^N, where N is ceil(log2(length(B_k+Added_Delay)));
      | Wr_En:
      |   Used to set behavior to read or write from b_k memory.
      |   Write: 1, Read: 0
      | 
      | Data_out:
      |   Output signal after processing. Set to sample time "System Time". Signed Fixed Point of size "Fixed Point Word Size". Zero-order hold.
      | Valid_out:
      |   Signal identifying when the output is a new processed value. Active high. Boolean.
      | RW_Dout:
      |   Returns the value stored in Wr_Addr, after a 1 System clock cycle delay.
      mask Display: disp(sprintf('Programmable Clock-Accelerated FIR\nMemory Used = %d bits \nFIR Length: %d \nClock Rate Needed = %d Hz', 2*2^FIR_SIZE*W_bits, 2^FIR_SIZE, maxRate)); port_label('input',1,'data'); port_label('input',2,'valid'); port_label('input',3,'Wr_Data'); port_label('input',4, 'RW_Addr'); port_label('input',5,'Wr_En'); port_label('output',1,'data'); port_label('output',2,'valid'); port_label('output',3,'RW_Dout');
  Static Upclocked FIR : Subsystem  mask(Static Upclocked FIR){b_k=[0.5,0.5], Ts=1/48000, Ts_system=1/96000, rotationDelay=0, W_bits=32, F_bits=28, maxRate=48000}
      mask prompts: b_k "B_k coefficients (vector)"; Ts "Sample Time"; Ts_system "System Time"; rotationDelay "Added Delay"; W_bits "Fixed Point Word Size"; F_bits "Fixed Point Frac Size"
      mask help:
      | This block is designed for a hardware implementation of an FIR filter. The main advantage is resource sharing by using a single multiply/add at an increased clock rate to multiply the b_k coefficients and sum the results.
      | The cost is a slightly increased amount of RAM used and the requirement that the system can run at data_rate*b_k_length, where b_k_length is rounded up to the nearest power of 2. The gains over a traditional FIR are a vastly decreased latency and logic resource usage.
      mask init:
      | FIR_SIZE = ceil(log2(length(b_k)+rotationDelay));
      | FIR_UPRATE = 2^FIR_SIZE;
      | firCoeff = zeros(1,FIR_UPRATE);
      | firCoeff(1:length(b_k)) = b_k;
      | maxRate = 1/(Ts/FIR_UPRATE);
      | 
      | set_param(gcb,'MaskDisplay',"disp(sprintf('Static Clock-Accelerated FIR\nMemory Used = %d bits \nFIR Length: %d\nClock Rate Needed = %d Hz', 2*2^FIR_SIZE*W_bits, 2^FIR_SIZE, maxRate)); port_label('input',1,'data'); port_label('input',2,'valid'); port_label('output',1,'data'); port_label('output',2,'valid');")
      mask Help:
      | This block is designed for a hardware implementation of an FIR filter. The main advantage is resource sharing by using a single multiply/add at an increased clock rate to multiply the b_k coefficients and sum the results.
      | The cost is a slightly increased amount of RAM used and the requirement that the system can run at data_rate*b_k_length, where b_k_length is rounded up to the nearest power of 2. The gains over a traditional FIR are a vastly decreased latency and logic resource usage.
      | 
      | An "Added Delay" option is included as a way to save resources when delaying the filtered signal. The b_k RAM is padded with 0s to round length up to a power of 2. Therefore, many faster cycles are completely uneccessary. Since many b_k's are 0, they can be rotated to align with inputs starting before the most recent, effectively delaying the output signal with 0 extra resources used. Useful for things like realigning a signal after multi-channel processing, or any other reason to delay the signal. If Added Delay would cause rotation to read from undesired coefficients (not 0), on startup the system will automatically increase the size of the table. This doubles the RAM used, so if using a b_k length at or near a power of 2, or if a very long delay is required, this may not be the most efficient option.
      | 
      | 
      | B_k's are defined on system start-up and cannot be changed during runtime.
      | 
      | ------------------
      | Mask Parameters
      | ------------------
      | 
      | B_k coefficients:
      |   FIR filter coefficients
      | Sample Time:
      |   Amount of time between valid pulses, when the input signal needs to be recognized.
      | System Time:
      |   Amount of time between system clock cycles. Can be the same as Sample Time if Valid_in is always 1.
      | Added Delay:
      |   Adds a N-sample delay to the output. Check Documentation Description for details.
      | Fixed Point Word/Frac Size:
      |   Word and Fractional bit size of input and table data type. Data input and b_k's are assumed to be the same data type.
      | 
      | ----------
      | Block I/O
      | ----------
      | 
      | Data_in:
      |   Input signal to be processed. Can be of any rate a direct multiple of "Sample rate". Signed Fixed Point of size "Fixed Point Word Size".
      | Valid_in:
      |  Trigger to show input signal should be written to signal memory of FIR RAM. Active high. Boolean.
      | 
      | Data_out:
      |   Output signal after processing. Set to sample time "System Time". Signed Fixed Point of size "Fixed Point Word Size". Zero-order hold.
      | Valid_out:
      |   Signal identifying when the output is a new processed value. Active high. Boolean.
      mask DialogControl b_k Tooltip: Filter Coefficients
      mask DialogControl Ts Tooltip: Ts
      mask DialogControl Ts_system Tooltip: Ts_system
      mask DialogControl rotationDelay Tooltip: An efficient way to realign signals
      mask DialogControl W_bits Tooltip: W_bits, size of Fixed Point word
      mask DialogControl F_bits Tooltip: F_bits, size of fractional component of word
      mask Display: disp(sprintf('Static Clock-Accelerated FIR\nMemory Used = %d bits \nFIR Length: %d\nClock Rate Needed = %d Hz', 2*2^FIR_SIZE*W_bits, 2^FIR_SIZE, maxRate)); port_label('input',1,'data'); port_label('input',2,'valid'); port_label('output',1,'data'); port_label('output',2,'valid');
  Variable Delay Block : Subsystem  mask(Variable Delay Block){maxDelay=2^4 -1}
      mask prompts: maxDelay "Maximum Delay"
      mask help:
      | A hardware-oriented implementation of a variable delay.
      | Provides a 0-latency selection of data history, where delay is an input port.
      mask init:
      | %% VARIABLE DELAY INIT SCRIPT
      | 
      | % Copyright 2020 Flat Earth Inc
      | %
      | % THE SOFTWARE IS PROVIDED "AS IS", WITHOUT WARRANTY OF ANY KIND, EXPRESS OR IMPLIED,
      | % INCLUDING BUT NOT LIMITED TO THE WARRANTIES OF MERCHANTABILITY, FITNESS FOR A PARTICULAR
      | % PURPOSE AND NONINFRINGEMENT. IN NO EVENT SHALL THE AUTHORS OR COPYRIGHT HOLDERS BE LIABLE
      | % FOR ANY CLAIM, DAMAGES OR OTHER LIABILITY, WHETHER IN AN ACTION OF CONTRACT, TORT OR OTHERWISE,
      | % ARISING FROM, OUT OF OR IN CONNECTION WITH THE SOFTWARE OR THE USE OR OTHER DEALINGS IN THE SOFTWARE.
      | %
      | % E. Bailey Galacci
      | % Flat Earth Inc
      | % 985 Technology Blvd
      | % Bozeman, MT 59718
      | % support@flatearthinc.com
      | 
      | % things to display: ram size, shift_delay
      | % things to figure out: ram size
      | 
      | % Identify RAM size needed
      | RAM_SIZE = ceil(log2(maxDelay+1));
      | 
      | %disp(sprintf('Variable Delay Block\nDelay Signal Width: %d\nRAM Size (Max Delay): %d', RAM_SIZE, 2^RAM_SIZE-1)) 
      | 
      | set_param(gcb,'MaskDisplay',"disp(sprintf('Variable Delay Block\nDelay Signal Width: %d\nRAM Size (Max Delay): %d', RAM_SIZE, 2^RAM_SIZE-1)); port_label('input',1,'Data_In'); port_label('input',2,'Data_Valid'); port_label('input',3,'Delay_Select'); port_label('output',1,'Data_Out');")
      mask Help:
      | ## Circular Buffer, Variable Delay
      | A hardware-oriented implementation of a variable delay.
      | Provides a zero-latency selection of data history, where delay is an input port.
      | 
      | The display shows Delay input signal width, as well as the maximum delay supported by the user's parameters.
      | 
      | ### Mask Parameters
      | 
      | - Maximum Delay
      |   Defines the maxmimum delay required by the user.
      |   Actual maximum delay (shown on the front) will be 2^N -1, where N = ceil(log2(maxDelay+1));
      |   This is for implementation reasons.
      | 
      | ### Block I/O
      | This section allows the user to drive the Simulink library blocks with input source signals and route the output signals.
      | 
      | #### Inputs:
      | Block input descriptions below.
      | - Data_In:
      |   Input signal. Size is automatically read during simulation or code generation.
      | - Data_Valid:
      |   Boolean. Set to 1 when input is valid, 0 otherwise.
      | - Delay_Select:
      |   Unsigned size N. Signals will be automatically converted to this size.
      |   Allows the user to select a desired delay for the block. Adjustable at any rate, regardless of Data_In rate.
      |   Always considered valid.
      | 
      |   A value of zero on this line effectively uses this block as a Zero-order hold until changed. Once set to any non-zero value,
      |   the output of the block will be the valid input from (Delay) samples ago, even if the Data_Valid signal is not asserted.
      |   Any value on this line greater than 2^N-1 will be truncated down to N bits.
      | 
      |   Note: It is highly recommended to use input signals all of the same clock rate. This will provide the most efficient VHDL code.
      |   The Data_Valid signal allows upclocking above the sample rate to support this.
      | 
      | #### Outputs:
      | Block output descriptions below.
      | 
      | - Data_Out:
      |   Delayed input data.
      mask Display: disp(sprintf('Variable Delay Block\nDelay Signal Width: %d\nRAM Size (Max Delay): %d', RAM_SIZE, 2^RAM_SIZE-1)); port_label('input',1,'Data_In'); port_label('input',2,'Data_Valid'); port_label('input',3,'Delay_Select'); port_label('output',1,'Data_Out');
